simulink model "model1"  (R2023a)
settings: Solver=ode4  StartTime=0.0  StopTime=10.0  FixedStep=1/216000  RelTol=1e-3
settings Model: Creator=tnt4  LastModifiedBy=tnt4
settings RTWCC: GPUComputeCapability=5.0

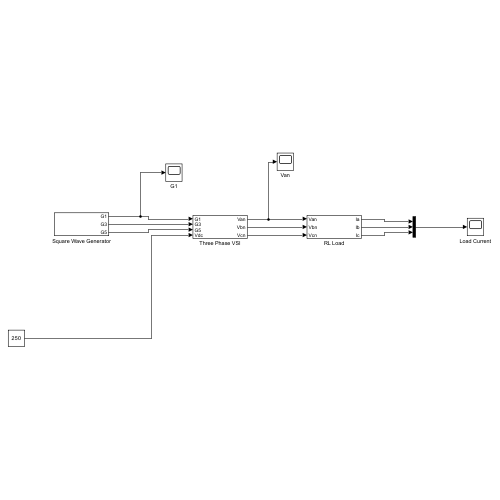
[thumbnail: Simulink's stored preview of the top-level diagram]
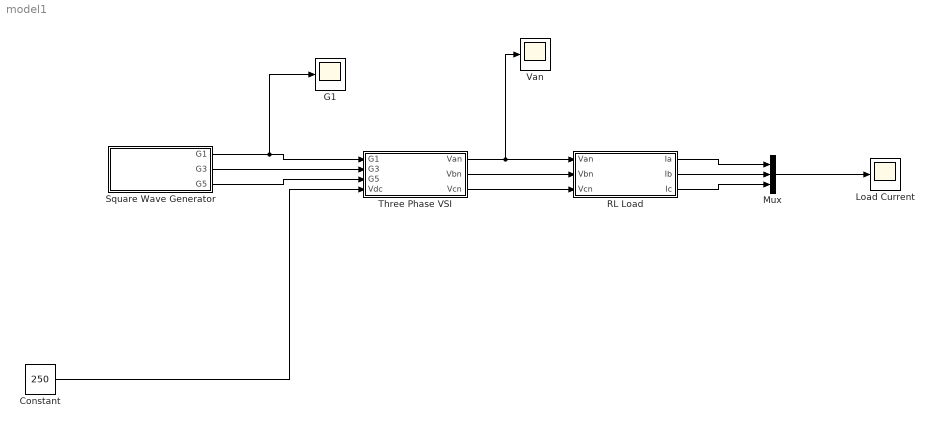
== system model1 ==
  Constant : Constant  Value=250
  G1 : Scope
  Load Current : Scope
  Mux : Mux  Inputs=3
  RL Load : Subsystem  mask{R_load=5, L_load=0.05}
      mask prompts: R_load "Resistance"; L_load "Inductance"
  Square Wave Generator : Subsystem  mask{Freq=60}
      mask prompts: Freq "Frequency (Hz)"
  Three Phase VSI : Subsystem
  Van : Scope
  wires:
  Square Wave Generator/1(G1) -> G1/1, Three Phase VSI/1(G1)
  Square Wave Generator/3(G5) -> Three Phase VSI/3(G5)
  Square Wave Generator/2(G3) -> Three Phase VSI/2(G3)
  Constant/1 -> Three Phase VSI/4(Vdc)
  Three Phase VSI/1(Van) -> Van/1, RL Load/1(Van)
  Three Phase VSI/2(Vbn) -> RL Load/2(Vbn)
  Three Phase VSI/3(Vcn) -> RL Load/3(Vcn)
  RL Load/1(Ia) -> Mux/1
  RL Load/2(Ib) -> Mux/2
  RL Load/3(Ic) -> Mux/3
  Mux/1 -> Load Current/1

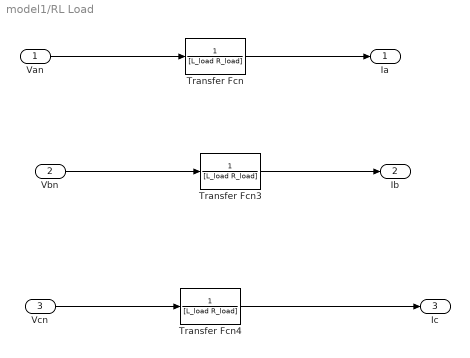
== system model1/RL Load ==
  Van : Inport
  Vbn : Inport  Port=2
  Vcn : Inport  Port=3
  Transfer Fcn : TransferFcn  Denominator=[L_load R_load]
  Transfer Fcn3 : TransferFcn  Denominator=[L_load R_load]
  Transfer Fcn4 : TransferFcn  Denominator=[L_load R_load]
  Ia : Outport
  Ib : Outport  Port=2
  Ic : Outport  Port=3
  wires:
  Transfer Fcn/1 -> Ia/1
  Van/1 -> Transfer Fcn/1
  Transfer Fcn3/1 -> Ib/1
  Vbn/1 -> Transfer Fcn3/1
  Vcn/1 -> Transfer Fcn4/1
  Transfer Fcn4/1 -> Ic/1

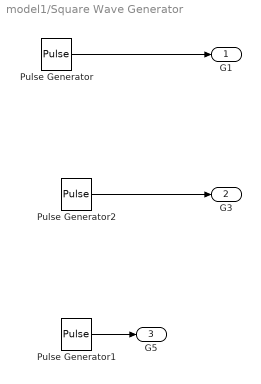
== system model1/Square Wave Generator ==
  Pulse Generator : DiscretePulseGenerator  PulseType=Time based  Period=1/Freq  PulseWidth=50
  Pulse Generator1 : DiscretePulseGenerator  PulseType=Time based  Period=1/Freq  PulseWidth=50  PhaseDelay=2/(3*Freq)
  Pulse Generator2 : DiscretePulseGenerator  PulseType=Time based  Period=1/Freq  PulseWidth=50  PhaseDelay=1/(3*Freq)
  G1 : Outport
  G3 : Outport  Port=2
  G5 : Outport  Port=3
  wires:
  Pulse Generator/1 -> G1/1
  Pulse Generator2/1 -> G3/1
  Pulse Generator1/1 -> G5/1

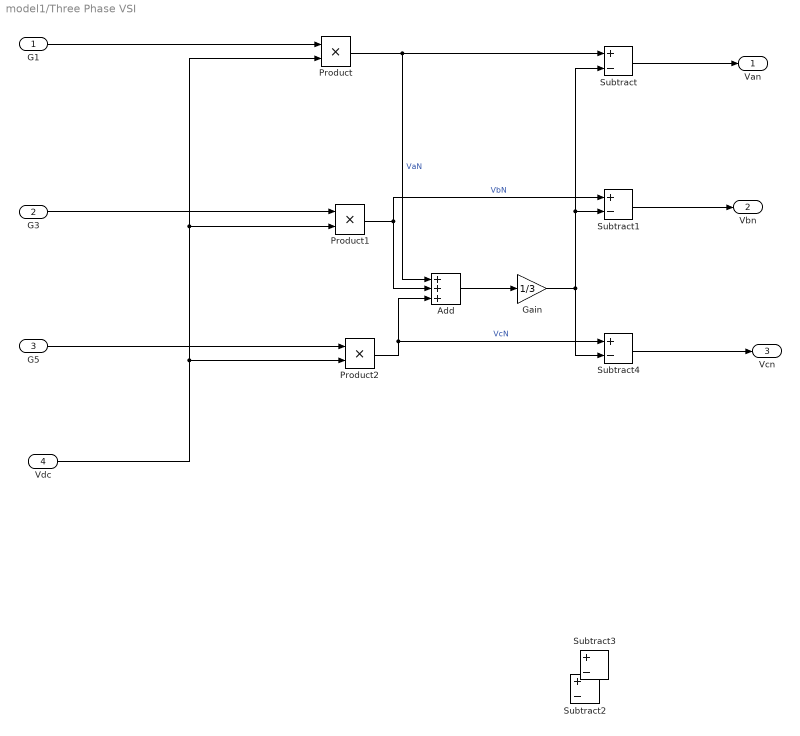
== system model1/Three Phase VSI ==
  G1 : Inport
  G3 : Inport  Port=2
  G5 : Inport  Port=3
  Vdc : Inport  Port=4
  Add : Sum  Inputs=+++
  Gain : Gain  Gain=1/3
  Product : Product
  Product1 : Product
  Product2 : Product
  Subtract{,1..4} (5 alike) : Sum  Inputs=+-
  Van : Outport
  Vbn : Outport  Port=2
  Vcn : Outport  Port=3
  wires:
  G1/1 -> Product/1
  G3/1 -> Product1/1
  G5/1 -> Product2/1
  Vdc/1 -> Product2/2, Product1/2, Product/2
  Product/1 -> Subtract/1, Add/1  "VaN"
  Product1/1 -> Add/2, Subtract1/1  "VbN"
  Product2/1 -> Add/3, Subtract4/1  "VcN"
  Add/1 -> Gain/1
  Gain/1 -> Subtract4/2, Subtract1/2, Subtract/2
  Subtract/1 -> Van/1
  Subtract1/1 -> Vbn/1
  Subtract4/1 -> Vcn/1
